simulink model "IonSatSimulationY"  (R2020b)
settings: Solver=ode3  StartTime=0.0  StopTime=t_sim  FixedStep=TimeStep  MaxStep=30  MinStep=.1  RelTol=1e-3
model workspace (MAT data in the model file):
  repartition_matrix : Simulink.Parameter (value not decoded)
  wheel_number : Simulink.Parameter (value not decoded)
values from neighbouring files (symbols this model uses):
  MODE = 2    [main_ADCS.m]    (also in main_ADCSv1.m)
  nmax = 2    [main_ADCS.m]    (also in main_ADCSv1.m)
  Use_IGRF = 1    [main_ADCS.m]    (also in main_ADCSv1.m)
  Use_IGRF_KF = 1    [main_ADCS.m]    (also in main_ADCSv1.m)
undefined symbols (not defined in the file or in its folder): att, AX, AY, AZ, AZES, Cdrag, CLS, Cmy, CRS, date, deg, DipoleMod, DiscIntNeverNeededParam, ESS, G, km, m, OGX, OGY, OGZ, orbit, OX, OY, OZ, rad, s, sat
libraries: aerolibutil x29, vrlib x26, aerolibconvert2 x15, simulink x10, sharedtransform x8, dspmathops x6, sharedutil x4, dspindex x3, aerolibobsolete x2, aerolibgravity2 x2, aerolibcelestial x2, dspstat3 x1
(part 4 of 4)

== matlab function IonSatSimulationY/Disturbance Torques /drag_torque/here we take care of the shadowing /If Action Subsystem/MATLAB Function ==
  data: G input; vorbit input; y output
function y = fcn(G, vorbit)
% les 4 points qui delimite le cadre 1
A=[0.17,0.11,0.05];%ok
B=[0.17,0.28,0.05];
C=[-0.17,0.28,0.05];
D=[-0.17,0.11,0.05];%ok


torque=[0,0,0];


%projection of B
pBy=0.11;
t=(pBy-B(2))/vorbit(2);
pBx=B(1)+t*vorbit(1);
pBz=B(3)+t*vorbit(3);

%projection of c
pCy=pBy;
pCx=C(1)+t*vorbit(1);%% because they have the same y
pCz=pBz;%%because of //
%vecteur directeur de notre droite
ux=A(1)-pBx;
uy=A(2)-pBy;%% zero we are in zx plan
uz=A(3)-pBz;
if pCz>-0.05
    if pBx<0.17
        
        if pBx>-0.17 %%we caculate(frcement pCx<-0.17)
            %pas
            N=100;%%%%%%%%%%%%%%%%%%%can be changed
            pas=ux/N;
            %integrale de rieman
            for i=0:N-1
                x=pBx+i*pas;
                t=(x-A(1))/ux;
                z=A(3)+t*uz;
                %geometric center for dA
                Gc=[x+(pas/2),pBy,(z-0.05)/2];
                Rs=Gc-G;
                torque= torque +cross(Rs,vorbit)*((z+0.05)*pas);
            end
            %the other surface
            Gc=[(pBx-0.17)/2,pBy,(pBz-0.05)/2];
            Rs=Gc-G;
            torque=torque+(pBx+0.17)*(pBz+0.05)*cross(Rs,vorbit);
        else
            %%we starte (la droite (ApB) coupe [segment]
            N=200;
            pas=0.34/N;
            
            for i=0:N-1
                x=-0.17+i*pas;
                t=(x-A(1))/ux;
                z=A(3)+t*uz;
                Gc=[x+(pas/2),pBy,(z-0.05)/2];
                Rs=Gc-G;
                torque= torque +cross(Rs,vorbit)*((z+0.05)*pas);
                
            end
            
            
            
        end
        
    elseif pCx<0.17 %%we konw already that pCx>-0.17
        %we calculate
        ux=D(1)-pCx;
        uy=D(2)-pCy;%%zero
        uz=D(3)-pCz;
        N=100;
        pas=ux/N;%negative always
       
        for i=0:N-1
            x=pCx+i*pas;
            t=(x-D(1))/ux;
            z=D(3)+t*uz;
            %geometric center for dA
            Gc=[x+(pas/2),pCy,(z-0.05)/2];
            Rs=Gc-G;
            torque= torque +cross(Rs,vorbit)*((z+0.05)*pas);
            
        end
        Gc=[(pCx+0.17)/2,pCy,(pCz-0.05)/2];
        Rs=Gc-G;
        torque=torque+(0.17-pCx)*(pCz+0.05)*cross(Rs,vorbit);
    else
        ux=D(1)-pCx;
        uy=D(2)-pCy;
        uz=D(3)-pCz;
        %we calculate(coupe droite segment)
        N=200;
        pas=-0.34/N;
     
        for i=0:N-1
            x=0.17+i*pas;
            t=(x-D(1))/ux;
            z=D(3)+t*uz;
            Gc=[x+(pas/2),pCy,(z-0.05)/2];
            Rs=Gc-G;
            torque= torque +cross(Rs,vorbit)*((z+0.05)*pas);
            
        end
        
    end
else
    %let Dprim Aprim to be like
    Dprim=[-0.17,0.11,-0.05];
    Aprim=[0.17,0.11,-0.05];
    if pBx<0.17
        ux=A(1)-pBx;
        uy=A(2)-pBy;
        uz=A(3)-pBz;
        %%%%
        ADpv=A-Dprim;
        %%%%%
        tprim=(pBz-A(3))/ADpv(3);
        %on compare
        xc=A(1)+tprim*ADpv(1);
        if pBx<xc%%%derriere suivant les x negative
            N=200;%%%%%%%%%%%%%%%%%%%can be changed
            pas=0.34/N;
            %integrale de rieman
            
            for i=0:N-1
                x=-0.17+i*pas;%%%intersection DDprim
                t=(x-A(1))/ux;
                z=A(3)+t*uz;
                %geometric center for dA
                Gc=[x+(pas/2),pBy,(z-0.05)/2];
                Rs=Gc-G;
                torque= torque +cross(Rs,vorbit)*((z+0.05)*pas);
            end
            
        else
            %we calculate%%%%%%%%%%problem(we can use diagonale)
            t=(-0.05-A(3))/uz;%%intersection DprimAprim
            x=A(1)+t*ux;
            N=100;%%%%%%%%%%%%%%%%%%%can be changed
            pas=(0.17-x)/N;
            %integrale de rieman
          
            for i=0:N-1
                x=x+i*pas;
                t=(x-A(1))/ux;
                z=A(3)+t*uz;
                %geometric center for dA
                Gc=[x+(pas/2),pBy,(z-0.05)/2];
                Rs=Gc-G;
                torque= torque +cross(Rs,vorbit)*((z+0.05)*pas);
            end
            
            
            
        end
        %%elseif pCx<0.17
        %we calculate
    else
        ux=D(1)-pCx;
        uy=D(2)-pCy;
        uz=D(3)-pCz;
        %%%%
        DApv=D-Aprim;
        %%%%%
        tprim=(pCz-A(3))/DApv(3);
        %on compare
        xc=D(1)+tprim*DApv(1);
        
        if pCx>xc
            N=200;%%%%%%%%%%%%%%%%%%%can be changed
            pas=-0.34/N;
            %integrale de rieman
            
            for i=0:N-1
                x=0.17+i*pas;
                t=(x-D(1))/ux;
                z=D(3)+t*uz;
                %geometric center for dA
                Gc=[x+(pas/2),pCy,(z-0.05)/2];
                Rs=Gc-G;
                torque= torque +cross(Rs,vorbit)*((z+0.05)*pas);
            end
            
        else
            %we calculate%%%%%%%%%%problem(we can use diagonale)
            t=(-0.05-D(3))/uz;
            x=D(1)+t*ux;
            N=100;%%%%%%%%%%%%%%%%%%%can be changed
            pas=(-0.17-x)/N;
            %integrale de rieman
           
            for i=0:N-1
                x=x+i*pas;
                t=(x-D(1))/ux;
                z=D(3)+t*uz;
                %geometric center for dA
                Gc=[x+(pas/2),pBy,(z-0.05)/2];
                Rs=Gc-G;
                torque= torque +cross(Rs,vorbit)*((z+0.05)*pas);
            end
            
            
            
        end
        
    end
    
end

y = torque;

== matlab function IonSatSimulationY/IGRF Computation block/ECI To LLA ==
  data: X_ECEF input; h output; lat output; long output
function [h, lat, long] = fcn(X_ECEF)
    h = 0;
    lat = 0;
    long = 0;
[lat, long, h] = ecef2geod(X_ECEF(1),X_ECEF(2),X_ECEF(3));

== matlab function IonSatSimulationY/Disturbance Torques /MATLAB Function2 ==
  data: u input; y output
function y = fcn(u)
y = u(6);

== matlab function IonSatSimulationY/Time propagator/UTC to JD ==
  data: Time_UTC input; JD output
function JD = fcn(Time_UTC)

% JD = juliandate(Time_UTC);
JD = Dt2jD(Time_UTC);

== matlab function IonSatSimulationY/Time propagator/JD to UTC ==
  data: JD input; Time_UTC output
function Time_UTC = fcn(JD)
    coder.extrinsic('datetime','datevec');
    Time_UTC = [0,0,0,0,0,0];
Time_UTC =  datevec(datetime(JD,'convertfrom','juliandate'));

== matlab function IonSatSimulationY/Subsystem/MATLAB Function ==
  data: u input; y output
function y = fcn(u)
boolean=0;
booleant=0;
if 5000<=u<=8000
    boolean=1;
end




y = booleant~=boolean;

== matlab function IonSatSimulationY/Disturbance Torques /drag_torque/here we take care of the shadowing /If Action Subsystem2/MATLAB Function ==
  data: G input; yy output; vorbit input
function yy = fcn(G, vorbit)
% les 4 points qui delimite le cadre 2
A=[0.17,0.11,0.05];%ok
B=[0.17,0.11,-0.05];
C=[-0.17,0.11,-0.05];
D=[-0.17,0.11,0.05];%ok


torque=[0,0,0];
%projection of B
pBz=0.05;
t=(pBz-B(3))/vorbit(3);
pBx=B(1)+t*vorbit(1);
pBy=B(2)+t*vorbit(2);

%projection of c
pCz=pBz;
pCx=C(1)+t*vorbit(1);%% 
pCy=pBy;%% because the projection is in this case //
%vecteur directeur de notre droite
ux=A(1)-pBx;
uy=A(2)-pBy;
uz=A(3)-pBz;

if pCy<0.28
    if pBx<0.17
        
        if pBx>-0.17 %%we caculate(frcement pCx<-0.17)
            %pas
            N=100;%%%%%%%%%%%%%%%%%%%can be changed
            pas=ux/N;
            %integrale de rieman
      
            for i=0:N-1
                x=pBx+i*pas;
                t=(x-A(1))/ux;
                y=A(2)+t*uy;
                %geometric center for dA
                Gc=[x+(pas/2),(0.28+y)/2,pBz];
                Rs=Gc-G;
                torque= torque +cross(Rs,vorbit)*((0.28-y)*pas);
            end
            %the other surface
            Gc=[(pBx-0.17)/2,(pBy+0.28)/2,pBz];
            Rs=Gc-G;
            torque=torque+(pBx+0.17)*(0.28-pBy)*cross(Rs,vorbit);
        else
            %%we calculate(la droite (ApB) coupe [segment]
            N=200;
            pas=0.34/N;
            
            for i=0:N-1
                x=-0.17+i*pas;
                t=(x-A(1))/ux;
                y=A(2)+t*uy;
                Gc=[x+(pas/2),(y+0.28)/2,pBz];
                Rs=Gc-G;
                torque= torque +cross(Rs,vorbit)*((0.28-y)*pas);
                
            end
            
            
            
        end
        
    elseif pCx<0.17 %%we konw already that pCx>-0.17
        %we calculate
        ux=D(1)-pCx;
        uy=D(2)-pCy;
        uz=D(3)-pCz;
        N=100;
        pas=ux/N;%negative always
       
        for i=0:N-1
            x=pCx+i*pas;
            t=(x-D(1))/ux;
            y=D(2)+t*uy;
            %geometric center for dA
            Gc=[x+(pas/2),(y+0.28)/2,pCz];
            Rs=Gc-G;
            torque= torque +cross(Rs,vorbit)*((0.28-y)*pas);
            
        end
        Gc=[(pCx+0.17)/2,(pCy+0.28)/2,pCz];
        Rs=Gc-G;
        torque=torque+(0.17-pCx)*(0.28-pCy)*cross(Rs,vorbit);
    else
        ux=D(1)-pCx;
        uy=D(2)-pCy;
        uz=D(3)-pCz;
        %we calculate(coupe droite segment)
        N=200;
        pas=-0.34/N;
     
        for i=0:N-1
            x=0.17+i*pas;
            t=(x-D(1))/ux;
            y=D(2)+t*uy;
            Gc=[x+(pas/2),(y+0.28)/2,pCz];
            Rs=Gc-G;
            torque= torque +cross(Rs,vorbit)*((0.28-y)*pas);
            
        end
        
    end
else
    %let Dprim Aprim to be like
    Dprim=[-0.17,0.28,0.05];
    Aprim=[0.17,0.28,0.05];
    if pBx<0.17
        ux=A(1)-pBx;
        uy=A(2)-pBy;
        uz=A(3)-pBz;
        %%%%
        ADpv=A-Dprim;
        %%%%%
        tprim=(pBy-A(2))/ADpv(2);
        %on compare
        xc=A(1)+tprim*ADpv(1);
        if pBx<xc%%%derriere suivant les x negative
            N=200;%%%%%%%%%%%%%%%%%%%can be changed
            pas=0.34/N;
            %integrale de rieman
            
            for i=0:N-1
                x=-0.17+i*pas;%%%intersection DDprim
                t=(x-A(1))/ux;
                y=A(2)+t*uy;
                %geometric center for dA
                Gc=[x+(pas/2),(y+0.28)/2,pBz];
                Rs=Gc-G;
                torque= torque +cross(Rs,vorbit)*((0.28-y)*pas);
            end
            
        else
            %we calculate%%%%%%%%%%problem(we can use diagonale)
            t=(0.28-A(2))/uy;%%intersection DprimAprim
            x=A(1)+t*ux;
            N=100;%%%%%%%%%%%%%%%%%%%can be changed
            pas=(0.17-x)/N;
            %integrale de rieman
          
            for i=0:N-1
                x=x+i*pas;
                t=(x-A(1))/ux;
                y=A(2)+t*uy;
                %geometric center for dA
                Gc=[x+(pas/2),(y+0.28)/2,pBz];
                Rs=Gc-G;
                torque= torque +cross(Rs,vorbit)*((0.28-y)*pas);
            end
            
            
            
        end
        %%elseif pCx<0.17
        %we calculate
    else
        ux=D(1)-pCx;
        uy=D(2)-pCy;
        uz=D(3)-pCz;
        %%%%
        DApv=D-Aprim;
        %%%%%
        tprim=(pCy-A(2))/DApv(2);
        %on compare
        xc=D(1)+tprim*DApv(1);
        
        if pCx>xc
            N=200;%%%%%%%%%%%%%%%%%%%can be changed
            pas=-0.34/N;
            %integrale de rieman
            
            for i=0:N-1
                x=0.17+i*pas;
                t=(x-D(1))/ux;
                y=D(2)+t*uy;
                %geometric center for dA
                Gc=[x+(pas/2),(y+0.28)/2,pCz];
                Rs=Gc-G;
                torque= torque +cross(Rs,vorbit)*((0.28-y)*pas);
            end
            
        else
            %we calculate%%%%%%%%%%problem(we can use diagonale)
            t=(0.28-D(2))/uy;
            x=D(1)+t*ux;
            N=100;%%%%%%%%%%%%%%%%%%%can be changed
            pas=(-0.17-x)/N;
            %integrale de rieman
           
            for i=0:N-1
                x=x+i*pas;
                t=(x-D(1))/ux;
                y=D(2)+t*uy;
                %geometric center for dA
                Gc=[x+(pas/2),(y+0.28)/2,pCz];
                Rs=Gc-G;
                torque= torque +cross(Rs,vorbit)*((0.28-y)*pas);
            end
            
            
            
        end
        
    end
    
end


yy = torque;
